simulink model "wj"  (R2022b)
settings: Solver=VariableStepAuto  StartTime=0.0  StopTime=10.0  RelTol=1e-3
settings Model: Creator=adlercohen  LastModifiedBy=adlercohen

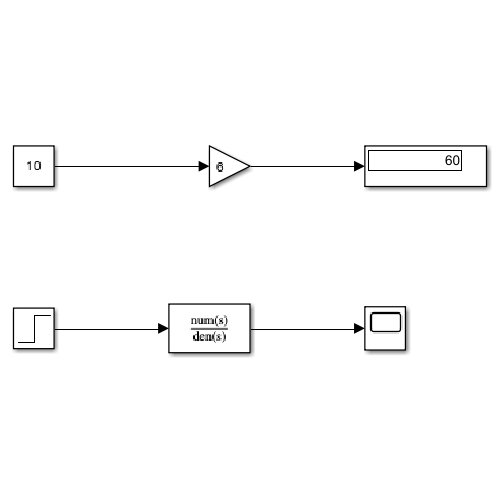
[thumbnail: Simulink's stored preview of the top-level diagram]
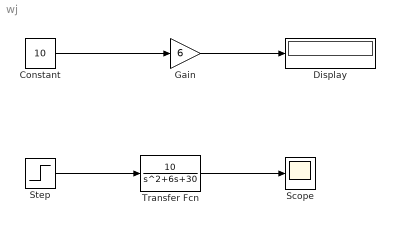
== system wj ==
  Constant : Constant  Value=10
  Display : Display
  Gain : Gain  Gain=6
  Scope : Scope
  Step : Step  Time=0  After=20  SampleTime=0
  Transfer Fcn : TransferFcn  Numerator=[10]  Denominator=[1 6 30]
  wires:
  Constant/1 -> Gain/1
  Gain/1 -> Display/1
  Step/1 -> Transfer Fcn/1
  Transfer Fcn/1 -> Scope/1
